simulink model "fftanalyzeri"  (R2012b)
settings: Solver=ode3  SolverMode=SingleTasking  StartTime=0.0  StopTime=20000  RelTol=1e-3
undefined symbols (not defined in the file or in its folder): pfb_coeff_gen_calc
undefined symbols (not defined in the file): fft_bin_flags_, magphmeanmem_, threshmem_
libraries: xbsIndex_r4 x9073, casper_library_misc x119, casper_library_flow_control x51, casper_library_delays x22, xps_library x10
(part 3 of 74)

== system fftanalyzeri/PulseDetector ==
  note: we take angle of 18.15. That is up to almost 4pi, or 4. normalixed by pi.
      | we want to nrmalize to +/-pi. So we keep buts 15 to 0, with bit 15 as a sign bit
      | This removes the 2pi jumps, keeping them around 0. We do not have
      | stuff around 2pi then stuff around 0-.
  note: Chan, din, dvldin can come on same clock.
      | we add puipe line delay for reading exp vals from the RAMs
  note: delauy for exp val ram read.
  note: Should be rams so we can save them...
  note: save current pylse bit, is_pulse, to ram, for this channel.
      | next time we read channel, we rememver if we are still reading a pulse
  note: Clear detected pulse
  note: rd en signal is a data valid signal, that will enable each part of the circult
  note: every time we switch which channel we are reading, we have to percuilate fresh data through this
      | whole circuit. it is 7 z's. so we have 7 clocks before we even know if there is a valid pulse or not.
      | The state machine controlling reading of the channel fifos must be able to wait for these 7 z's before it switches
      | to a new channel to read. We will generate a done sugnal telling that the pulse detection is done, and we are
      | free to readout a new channel fifo.
  note: rd signal aligend w/ output of pulse detector
  note: read sigakl delay- accounts for labntecy in the calcs
  note: 1 of pulse
      | 0 of no pulse
  note: Now we cpmpare  LLD with  the computed val
      | of 2 real samples, 2 im samples w/
      | DC offsets removed
  note: Add delayed sig w/ siang.
      | This does filtering by taking
      | two re samples and two im
      | samples and adding all
  note: Delay bu on sample
  note: Annd re and im together
  note: Take abs value to get all
      | piositive data
  note: Take out the expected value
      | or any DC offset
  note: delauy for exp val ram read.
  dvld_in : Inport
  din : Inport  Port=2
  clear : Inport  Port=3
  en : Inport  Port=4
  chan : Inport  Port=5
  savepulsestate : Inport  Port=6
  Absolute : xbsIndex_r4/Absolute  precision=User Defined  arith_type=Unsigned  n_bits=18  bin_pt=16  quantization=Truncate  overflow=Wrap  en=on  latency=1  dbl_ovrd=off  block_type=abs
  Absolute1 : xbsIndex_r4/Absolute  precision=User Defined  arith_type=Unsigned  n_bits=18  bin_pt=16  quantization=Truncate  overflow=Wrap  en=on  latency=1  dbl_ovrd=off  block_type=abs
  AddSub2 : xbsIndex_r4/AddSub  mode=Subtraction  use_carryin=off  use_carryout=off  en=on  latency=1  precision=User Defined  arith_type="Signed  (2's comp)"  n_bits=18  bin_pt=16  quantization=Truncate  overflow=Wrap  dbl_ovrd=off  use_behavioral_HDL=off  hw_selection=Fabric  pipelined=off  block_type=addsub
  AddSub3 : xbsIndex_r4/AddSub  mode=Subtraction  use_carryin=off  use_carryout=off  en=on  latency=1  precision=User Defined  arith_type="Signed  (2's comp)"  n_bits=18  bin_pt=16  quantization=Truncate  overflow=Wrap  dbl_ovrd=off  use_behavioral_HDL=off  hw_selection=Fabric  pipelined=off  block_type=addsub
  AddSub4 : xbsIndex_r4/AddSub  mode=Addition  use_carryin=off  use_carryout=off  en=on  latency=1  precision=User Defined  arith_type="Signed  (2's comp)"  n_bits=18  bin_pt=16  quantization=Truncate  overflow=Wrap  dbl_ovrd=off  use_behavioral_HDL=off  hw_selection=Fabric  pipelined=off  block_type=addsub
  AddSub5 : xbsIndex_r4/AddSub  mode=Addition  use_carryin=off  use_carryout=off  en=on  latency=1  precision=User Defined  arith_type="Signed  (2's comp)"  n_bits=19  bin_pt=16  quantization=Truncate  overflow=Wrap  dbl_ovrd=off  use_behavioral_HDL=off  hw_selection=Fabric  pipelined=off  block_type=addsub
  Delay{,6..8} (4 alike) : xbsIndex_r4/Delay  rst=on  infoeditControl=Selection of Reset will increase slice count due to use of real FFs and instead of SRLs  en=on  latency=1  dbl_ovrd=off  reg_retiming=off  block_type=delay
  Delay1 : xbsIndex_r4/Delay  rst=off  infoeditControl=Selection of Reset will increase slice count due to use of real FFs and instead of SRLs  en=on  latency=7  dbl_ovrd=off  reg_retiming=off  block_type=delay
  Delay2 : xbsIndex_r4/Delay  rst=on  infoeditControl=Selection of Reset will increase slice count due to use of real FFs and instead of SRLs  en=on  latency=5  dbl_ovrd=off  reg_retiming=off  block_type=delay
  Delay3 : xbsIndex_r4/Delay  rst=off  infoeditControl=Selection of Reset will increase slice count due to use of real FFs and instead of SRLs  en=on  latency=1  dbl_ovrd=off  reg_retiming=off  block_type=delay
  Delay4 : xbsIndex_r4/Delay  rst=off  infoeditControl=Selection of Reset will increase slice count due to use of real FFs and instead of SRLs  en=on  latency=1  dbl_ovrd=off  reg_retiming=off  block_type=delay
  Delay5 : xbsIndex_r4/Delay  rst=off  infoeditControl=Selection of Reset will increase slice count due to use of real FFs and instead of SRLs  en=off  latency=5  dbl_ovrd=off  reg_retiming=off  block_type=delay
  From Workspace2 : FromWorkspace  VariableName=PulseDetector_pulselength  SampleTime=1  Interpolate=off  OutputAfterFinalValue=Holding final value
  Gateway Out{,1..7} (8 alike) : xbsIndex_r4/Gateway Out  inherit_from_input=off  hdl_port=on  timing_constraint=None  locs_specified=off  LOCs={}  UseAsDAC=off  DACChannel='1'  block_type=gatewayout
  Logical : xbsIndex_r4/Logical  logical_function=OR  inputs=2  en=off  latency=0  precision=Full  arith_type=Unsigned  n_bits=16  bin_pt=0  align_bp=on  dbl_ovrd=off  block_type=logical
  Logical1 : xbsIndex_r4/Logical  logical_function=OR  inputs=2  en=off  latency=0  precision=Full  arith_type=Unsigned  n_bits=16  bin_pt=0  align_bp=on  dbl_ovrd=off  block_type=logical
  Logical{2..5} (4 alike) : xbsIndex_r4/Logical  logical_function=AND  inputs=2  en=off  latency=0  precision=Full  arith_type=Unsigned  n_bits=16  bin_pt=0  align_bp=on  dbl_ovrd=off  block_type=logical
  Normalize180_ : Subsystem
  Normalize180_1 : Subsystem
  PulseLenCounter : xbsIndex_r4/Counter  cnt_type=Free Running  cnt_to=0  operation=Down  start_count=0  cnt_by_val=1  arith_type=Unsigned  n_bits=8  bin_pt=0  load_pin=on  rst=on  en=on  explicit_period=on  period=1  dbl_ovrd=off  use_behavioral_HDL=off  implementation=Fabric  block_type=counter
  PulseLength : xbsIndex_r4/Register  init=0  rst=on  en=on  dbl_ovrd=off  block_type=register
  Register1 : xbsIndex_r4/Register  init=0  rst=off  en=on  dbl_ovrd=off  block_type=register
  Relational : xbsIndex_r4/Relational  mode=a>b  en=off  latency=0  dbl_ovrd=off  block_type=relational
  Relational1 : xbsIndex_r4/Relational  mode=a!=b  en=off  latency=0  dbl_ovrd=off  block_type=relational
  bits_31_16_ : xbsIndex_r4/Slice  nbits=16  boolean_output=off  mode=Lower Bit Location + Width  bit1=0  base1=MSB of Input  bit0=16  base0=LSB of Input  dbl_ovrd=off  block_type=slice
  bool_ : xbsIndex_r4/Constant  const=0  gui_display_data_type=Boolean  arith_type=Boolean  n_bits=16  bin_pt=14  preci_type=Single  exp_width=8  frac_width=24  explicit_period=on  period=1  equ=P=C  opselect=C  inp2=PCIN>>17  opr=+  inp1=P  carry=CIN  dbl_ovrd=off  block_type=constant
  bool_6 : xbsIndex_r4/Constant  const=0  gui_display_data_type=Boolean  arith_type=Boolean  n_bits=16  bin_pt=14  preci_type=Single  exp_width=8  frac_width=24  explicit_period=on  period=1  equ=P=C  opselect=C  inp2=PCIN>>17  opr=+  inp1=P  carry=CIN  dbl_ovrd=off  block_type=constant
  bool_7 : xbsIndex_r4/Constant  const=1  gui_display_data_type=Boolean  arith_type=Boolean  n_bits=16  bin_pt=14  preci_type=Single  exp_width=8  frac_width=24  explicit_period=on  period=1  equ=P=C  opselect=C  inp2=PCIN>>17  opr=+  inp1=P  carry=CIN  dbl_ovrd=off  block_type=constant
  buts_15_0_ : xbsIndex_r4/Slice  nbits=16  boolean_output=off  mode=Lower Bit Location + Width  bit1=0  base1=MSB of Input  bit0=0  base0=LSB of Input  dbl_ovrd=off  block_type=slice
  buts_17_0_ : xbsIndex_r4/Slice  nbits=18  boolean_output=off  mode=Lower Bit Location + Width  bit1=0  base1=MSB of Input  bit0=0  base0=LSB of Input  dbl_ovrd=off  block_type=slice
  buts_7_0_1 : xbsIndex_r4/Slice  nbits=8  boolean_output=off  mode=Lower Bit Location + Width  bit1=0  base1=MSB of Input  bit0=0  base0=LSB of Input  dbl_ovrd=off  block_type=slice
  c2polar_ : Subsystem
  i16_13_2 : xbsIndex_r4/Reinterpret  force_arith_type=on  arith_type="Signed  (2's comp)"  force_bin_pt=on  bin_pt=13  block_type=reinterpret
  i16_14_1 : xbsIndex_r4/Reinterpret  force_arith_type=on  arith_type="Signed  (2's comp)"  force_bin_pt=on  bin_pt=14  block_type=reinterpret
  i18_16_3 : xbsIndex_r4/Reinterpret  force_arith_type=on  arith_type="Signed  (2's comp)"  force_bin_pt=on  bin_pt=16  block_type=reinterpret
  lsb8_ : xbsIndex_r4/Slice  nbits=8  boolean_output=off  mode=Lower Bit Location + Width  bit1=0  base1=MSB of Input  bit0=0  base0=LSB of Input  dbl_ovrd=off  block_type=slice
  meanmagph32_ : Subsystem  Tag=xps:bram  AncestorBlock=xps_library/Shared BRAM  mask{arith_type=Unsigned, addr_width=10, data_width=32, reg_prim_output=off, reg_core_output=off, optimization=Minimum_Area, data_bin_pt=0, init_vals=magphmeanmem_, sample_rate=1}
      mask prompts: arith_type "Output Data Type"; addr_width "Address width"; data_width "Data Width"; reg_prim_output "Register Primitive Output"; reg_core_output "Register Core Output"; data_bin_pt "Data Binary Point"; init_vals "Initial values (simulation only)"; sample_rate "Sample rate"
      mask init:
      | shared_bram_mask;
      mask TypeOptions arith_type: Unsigned | Signed  (2's comp)
      mask TypeOptions data_width: 8 | 16 | 32 | 64 | 128
      mask TypeOptions optimization: Minimum_Area | Low_Power
  pulseDetScope : Scope  NumInputPorts=8
      settings: YMin=-5~-5~-5~-5~-5~-5~-5~-5  YMax=5~5~5~5~5~5~5~5  SaveName=fsmdata2
  pulselength : Subsystem  Tag=xps:sw_reg  AncestorBlock=xps_library/software register  mask{numios=1, io_dir=From Processor, io_delay=0, sample_period=1, name1=reg, bitwidth1=32, arith_type1=Unsigned, bin_pt1=0}
      mask prompts: numios "Num I/Os"; io_dir "I/O direction"; io_delay "I/O delay"; sample_period "Sample period"; name1 "Name"; bitwidth1 "Bitwidth"; arith_type1 "Type"; bin_pt1 "Binary pt"
      mask init:
      | swreg_init(gcb);
      mask Callback numios: t = timer('StartDelay', 0.1); t.TimerFcn = {@swreg_cb, gcb}; start(t);
      mask TypeOptions io_dir: To Processor | From Processor
      mask Callback io_dir:
      | a = get_param(gcb, 'MaskEnables');
      | if strcmp(get_param(gcb, 'io_dir'), 'To Processor'),
      | a(4) = {'off'};
      | else
      | a(4) = {'on'};
      | end
      | set_param(gcb, 'MaskEnables', a);
      mask TypeOptions arith_type1: Unsigned | Signed  (2's comp) | Boolean
      mask Callback arith_type1:
      | a = get_param(gcb, 'MaskEnables');
      | if strcmp(get_param(gcb, 'arith_type1'), 'Boolean'),
      | set_param(gcb, 'bitwidth1', '1');
      | set_param(gcb, 'bin_pt1', '0');
      | a(6) = {'off'};
      | a(8) = {'off'};
      | else
      | a(6) = {'on'};
      | a(8) = {'on'};
      | end
      | set_param(gcb, 'MaskEnables', a);
  pulsestateRAM : xbsIndex_r4/Single Port RAM  depth=256  initVector=zeros(1,256)  distributed_mem=Block RAM  write_mode=Read After Write  rst=off  init_reg=0  en=off  latency=1  dbl_ovrd=off  optimize=Area  use_rpm=on  block_type=spram
  thresh32_1 : Subsystem  Tag=xps:bram  AncestorBlock=xps_library/Shared BRAM  mask{arith_type=Unsigned, addr_width=10, data_width=32, reg_prim_output=off, reg_core_output=off, optimization=Minimum_Area, data_bin_pt=0, init_vals=threshmem_, sample_rate=1}
      mask prompts: arith_type "Output Data Type"; addr_width "Address width"; data_width "Data Width"; reg_prim_output "Register Primitive Output"; reg_core_output "Register Core Output"; data_bin_pt "Data Binary Point"; init_vals "Initial values (simulation only)"; sample_rate "Sample rate"
      mask init:
      | shared_bram_mask;
      mask TypeOptions arith_type: Unsigned | Signed  (2's comp)
      mask TypeOptions data_width: 8 | 16 | 32 | 64 | 128
      mask TypeOptions optimization: Minimum_Area | Low_Power
  ui8_1 : xbsIndex_r4/Constant  const=0  gui_display_data_type=Fixed-point  arith_type=Unsigned  n_bits=8  bin_pt=0  preci_type=Single  exp_width=8  frac_width=24  explicit_period=on  period=1  equ=P=C  opselect=C  inp2=PCIN>>17  opr=+  inp1=P  carry=CIN  dbl_ovrd=off  block_type=constant
  uint32_ : xbsIndex_r4/Constant  const=0  gui_display_data_type=Fixed-point  arith_type=Unsigned  n_bits=32  bin_pt=0  preci_type=Single  exp_width=8  frac_width=24  explicit_period=on  period=1  equ=P=C  opselect=C  inp2=PCIN>>17  opr=+  inp1=P  carry=CIN  dbl_ovrd=off  block_type=constant
  datadly : Outport
  dvld_out : Outport  Port=2
  busy : Outport  Port=3
  pulse : Outport  Port=4
  detect : Outport  Port=5
  savedpulsestate : Outport  Port=6
  wires:
  Register1/1 -> AddSub5/2
  [magExpVal] -> AddSub2/2
  [phaseExpVal] -> Gateway Out2/1, AddSub3/2
  Delay8/1 -> detect/1, Logical/1, PulseLenCounter/1, Gateway Out7/1
  AddSub2/1 -> Absolute/1
  ui8_1/1 -> Relational1/1
  din/1 -> c2polar_/1(c), Delay1/1
  Absolute/1 -> AddSub4/1
  AddSub3/1 -> Normalize180_1/1(In1), Gateway Out3/1
  Absolute1/1 -> AddSub4/2, Gateway Out4/1
  Delay/1 -> Logical4/1, dvld_out/1, Logical1/1
  AddSub4/1 -> Gateway Out5/1, AddSub5/1, Register1/1
  PulseLenCounter/1 -> Relational1/2
  bool_7/1 -> PulseLength/3
  Delay5/1 -> Relational/2
  Delay1/1 -> datadly/1
  dvld_in/1 -> Delay2/1
  Relational1/1 -> Logical/2, Delay7/1
  bool_6/1 -> PulseLength/2
  AddSub5/1 -> Gateway Out6/1, Relational/1
  [pls_thresh] -> Delay5/1
  Logical1/1 -> busy/1
  Delay6/1 -> Logical2/1, Delay/1
  clear/1 -> Delay2/2, Delay/2, Delay6/2, Delay8/2, PulseLenCounter/3, Delay7/2
  Delay7/1 -> [is_pulse], pulse/1, Logical1/2
  Relational/1 -> Delay8/1
  PulseLength/1 -> PulseLenCounter/2
  en/1 -> [enable]
  [enable] -> Delay3/2, Delay2/3, Delay1/2, Delay/3, Delay6/3
  [enable] -> AddSub4/3, Absolute/2, Absolute1/2, AddSub2/3, AddSub3/3
  [enable] -> Register1/2
  Logical2/1 -> Delay8/3
  [enable] -> Logical2/2
  Logical3/1 -> PulseLenCounter/4
  Logical/1 -> Logical3/1
  [enable] -> Logical3/2
  Logical4/1 -> Delay7/3
  [enable] -> Logical4/2
  Delay2/1 -> Logical5/1, Delay6/1
  [enable] -> Logical5/2
  Logical5/1 -> AddSub5/3
  savepulsestate/1 -> pulsestateRAM/3
  [is_pulse] -> pulsestateRAM/2
  pulsestateRAM/1 -> savedpulsestate/1
  Delay3/1 -> AddSub2/1
  Delay4/1 -> Gateway Out1/1, AddSub3/1
  [enable] -> Delay4/2
  lsb8_/1 -> thresh32_1/1(addr), meanmagph32_/1(addr), pulsestateRAM/1
  c2polar_/2(phase) -> Gateway Out/1, Normalize180_/1(In1)
  c2polar_/1(power) -> Delay3/1
  pulselength/1(in_reg) -> buts_7_0_1/1
  From Workspace2/1 -> pulselength/1(sim_reg)
  buts_7_0_1/1 -> [pls_len]
  [pls_len] -> PulseLength/1
  Gateway Out/1 -> pulseDetScope/1
  Gateway Out1/1 -> pulseDetScope/2
  Gateway Out2/1 -> pulseDetScope/3
  Gateway Out3/1 -> pulseDetScope/4
  Gateway Out4/1 -> pulseDetScope/5
  Gateway Out5/1 -> pulseDetScope/6
  Gateway Out6/1 -> pulseDetScope/7
  Gateway Out7/1 -> pulseDetScope/8
  chan/1 -> lsb8_/1
  buts_15_0_/1 -> i16_14_1/1
  bits_31_16_/1 -> i16_13_2/1
  buts_17_0_/1 -> i18_16_3/1
  i16_14_1/1 -> [magExpVal]
  i16_13_2/1 -> [phaseExpVal]
  meanmagph32_/1(data_out) -> buts_15_0_/1, bits_31_16_/1
  i18_16_3/1 -> [pls_thresh]
  bool_/1 -> thresh32_1/3(we), meanmagph32_/3(we)
  thresh32_1/1(data_out) -> buts_17_0_/1
  uint32_/1 -> thresh32_1/2(data_in), meanmagph32_/2(data_in)
  Normalize180_/1(Out1) -> Delay4/1
  Normalize180_1/1(Out1) -> Absolute1/1

== system fftanalyzeri/RWen ==
  sim_reg : Inport
  fftanalyzeri_RWen_user_data_out : xbsIndex_r4/Gateway In  gui_display_data_type=Fixed-point  arith_type=Unsigned  n_bits=32  bin_pt=0  preci_type=Single  exp_width=8  frac_width=24  quantization="Round  (unbiased: +/- Inf)"  overflow=Saturate  period=1  dbl_ovrd=off  timing_constraint=None  locs_specified=off  LOCs={}  UseAsADC=off  ADCChannel='1'  inherit_from_input=off  hdl_port=on  block_type=gatewayin
  io_delay : xbsIndex_r4/Delay  rst=off  infoeditControl=Selection of Reset will increase slice count due to use of real FFs and instead of SRLs  en=off  latency=0  dbl_ovrd=off  reg_retiming=on  block_type=delay
  reint1 : xbsIndex_r4/Reinterpret  force_arith_type=on  arith_type=Unsigned  force_bin_pt=on  bin_pt=0  block_type=reinterpret
  slice_reg : xbsIndex_r4/Slice  nbits=32  boolean_output=off  mode=Lower Bit Location + Width  bit1=0  base1=MSB of Input  bit0=0  base0=LSB of Input  dbl_ovrd=off  block_type=slice
  in_reg : Outport
  wires:
  fftanalyzeri_RWen_user_data_out/1 -> io_delay/1
  sim_reg/1 -> fftanalyzeri_RWen_user_data_out/1
  io_delay/1 -> slice_reg/1
  slice_reg/1 -> reint1/1
  reint1/1 -> in_reg/1

== system fftanalyzeri/RectToPolar ==
  note: shoudl be same delay as cordic. if it takes 18 clocks to go
      | through cordic, it hould be 18 here.
  note: input re and im.
      | output magnitude and phase
      | phase is from 0 to 2, where 2 is 2pi.
      | put as complex number where im part is actuaol phase
      | 18 bit data, phase in NOT radians but mult of pi.
      | phse/pi is output. Translate alg. where imagine we translate the vector (k,0)
      | phase is how much we rotated the cord. to make the 0.
  dvld_in : Inport
  cmplx_din : Inport  Port=2
  chan : Inport  Port=3
  "CORDIC 4.0 " : xbsIndex_r4/CORDIC 4.0   functional_selection=Translate  architectural_configuration=Parallel  pipelining_mode=Maximum  data_format=SignedFraction  phase_format=Scaled_Radians  output_width=18  round_mode=Truncate  iterations=0  precision=0  coarse_rotation=on  compensation_scaling=Embedded_Multiplier  ce=off  sclr=off  nd=on  rdy=on  x_out=on  y_out=off  phase_output=on  register_inputs=true  register_outputs=true  ipcore_usecache=true  ipcore_useipmodelcache=true  ipcore_verbose=false  wrapper_available=true  ip_name=CORDIC  ip_version=4.0  dsptool_ready=true  port_translation_map={ 'ce' => 'en', 'sclr' => 'rst' }  structural_sim=false  block_type=cordic_v4_0
  Delay : xbsIndex_r4/Delay  rst=off  infoeditControl=Selection of Reset will increase slice count due to use of real FFs and instead of SRLs  en=off  latency=25  dbl_ovrd=off  reg_retiming=off  block_type=delay
  Gateway Out{1..4,34..37} (8 alike) : xbsIndex_r4/Gateway Out  inherit_from_input=off  hdl_port=on  timing_constraint=None  locs_specified=off  LOCs={}  UseAsDAC=off  DACChannel='1'  block_type=gatewayout
  c_to_ri3 : casper_library_misc/c_to_ri  n_bits=18  bin_pt=16
      settings: AttributesFormatString=18_16 r/i
  i18_16_1 : xbsIndex_r4/Assert  assert_type=on  type_source=Explicitly  gui_display_data_type=Fixed-point  arith_type="Signed  (2's comp)"  n_bits=18  bin_pt=16  preci_type=Single  exp_width=8  frac_width=24  assert_rate=off  rate_source=Explicitly  period=1  output_port=on  block_type=assert
  i18_16_2 : xbsIndex_r4/Assert  assert_type=on  type_source=Explicitly  gui_display_data_type=Fixed-point  arith_type="Signed  (2's comp)"  n_bits=18  bin_pt=16  preci_type=Single  exp_width=8  frac_width=24  assert_rate=off  rate_source=Explicitly  period=1  output_port=on  block_type=assert
  rect2polar : Scope  NumInputPorts=8
      settings: YMin=-5~-5~-5~-5~-5~-5~-5~-5  YMax=5~5~5~5~5~5~5~5  SaveName=fsmdata10
  ri_to_c : casper_library_misc/ri_to_c
  dvld_out : Outport
  cmplx_dout : Outport  Port=2
  chandly : Outport  Port=3
  wires:
  c_to_ri3/2 -> Gateway Out37/1, i18_16_1/1
  dvld_in/1 -> Gateway Out3/1, "CORDIC 4.0 "/3
  c_to_ri3/1 -> Gateway Out36/1, i18_16_2/1
  ri_to_c/1 -> cmplx_dout/1
  "CORDIC 4.0 "/3 -> Gateway Out4/1, dvld_out/1
  "CORDIC 4.0 "/1 -> Gateway Out34/1, ri_to_c/1
  "CORDIC 4.0 "/2 -> Gateway Out35/1, ri_to_c/2
  i18_16_2/1 -> "CORDIC 4.0 "/1
  i18_16_1/1 -> "CORDIC 4.0 "/2
  cmplx_din/1 -> c_to_ri3/1
  Delay/1 -> Gateway Out2/1, chandly/1
  chan/1 -> Gateway Out1/1, Delay/1
  Gateway Out36/1 -> rect2polar/1
  Gateway Out37/1 -> rect2polar/2
  Gateway Out34/1 -> rect2polar/3
  Gateway Out35/1 -> rect2polar/4
  Gateway Out3/1 -> rect2polar/5
  Gateway Out4/1 -> rect2polar/6
  Gateway Out1/1 -> rect2polar/7
  Gateway Out2/1 -> rect2polar/8

== system fftanalyzeri/RectToPolar1 ==
  note: shoudl be same delay as cordic. if it takes 18 clocks to go
      | through cordic, it hould be 18 here.
  note: input re and im.
      | output magnitude and phase
      | phase is from 0 to 2, where 2 is 2pi.
      | put as complex number where im part is actuaol phase
      | 18 bit data, phase in NOT radians but mult of pi.
      | phse/pi is output. Translate alg. where imagine we translate the vector (k,0)
      | phase is how much we rotated the cord. to make the 0.
  dvld_in : Inport
  cmplx_din : Inport  Port=2
  chan : Inport  Port=3
  "CORDIC 4.0 " : xbsIndex_r4/CORDIC 4.0   functional_selection=Translate  architectural_configuration=Parallel  pipelining_mode=Maximum  data_format=SignedFraction  phase_format=Scaled_Radians  output_width=18  round_mode=Truncate  iterations=0  precision=0  coarse_rotation=on  compensation_scaling=Embedded_Multiplier  ce=off  sclr=off  nd=on  rdy=on  x_out=on  y_out=off  phase_output=on  register_inputs=true  register_outputs=true  ipcore_usecache=true  ipcore_useipmodelcache=true  ipcore_verbose=false  wrapper_available=true  ip_name=CORDIC  ip_version=4.0  dsptool_ready=true  port_translation_map={ 'ce' => 'en', 'sclr' => 'rst' }  structural_sim=false  block_type=cordic_v4_0
  Delay : xbsIndex_r4/Delay  rst=off  infoeditControl=Selection of Reset will increase slice count due to use of real FFs and instead of SRLs  en=off  latency=25  dbl_ovrd=off  reg_retiming=off  block_type=delay
  c_to_ri3 : casper_library_misc/c_to_ri  n_bits=18  bin_pt=16
      settings: AttributesFormatString=18_16 r/i
  i18_16_1 : xbsIndex_r4/Assert  assert_type=on  type_source=Explicitly  gui_display_data_type=Fixed-point  arith_type="Signed  (2's comp)"  n_bits=18  bin_pt=16  preci_type=Single  exp_width=8  frac_width=24  assert_rate=off  rate_source=Explicitly  period=1  output_port=on  block_type=assert
  i18_16_2 : xbsIndex_r4/Assert  assert_type=on  type_source=Explicitly  gui_display_data_type=Fixed-point  arith_type="Signed  (2's comp)"  n_bits=18  bin_pt=16  preci_type=Single  exp_width=8  frac_width=24  assert_rate=off  rate_source=Explicitly  period=1  output_port=on  block_type=assert
  ri_to_c : casper_library_misc/ri_to_c
  dvld_out : Outport
  cmplx_dout : Outport  Port=2
  chandly : Outport  Port=3
  wires:
  c_to_ri3/2 -> i18_16_1/1
  dvld_in/1 -> "CORDIC 4.0 "/3
  c_to_ri3/1 -> i18_16_2/1
  ri_to_c/1 -> cmplx_dout/1
  "CORDIC 4.0 "/3 -> dvld_out/1
  "CORDIC 4.0 "/1 -> ri_to_c/1
  "CORDIC 4.0 "/2 -> ri_to_c/2
  i18_16_2/1 -> "CORDIC 4.0 "/1
  i18_16_1/1 -> "CORDIC 4.0 "/2
  cmplx_din/1 -> c_to_ri3/1
  Delay/1 -> chandly/1
  chan/1 -> Delay/1

== system fftanalyzeri/RectToPolar2 ==
  note: shoudl be same delay as cordic. if it takes 18 clocks to go
      | through cordic, it hould be 18 here.
  note: input re and im.
      | output magnitude and phase
      | phase is from 0 to 2, where 2 is 2pi.
      | put as complex number where im part is actuaol phase
      | 18 bit data, phase in NOT radians but mult of pi.
      | phse/pi is output. Translate alg. where imagine we translate the vector (k,0)
      | phase is how much we rotated the cord. to make the 0.
  dvld_in : Inport
  cmplx_din : Inport  Port=2
  chan : Inport  Port=3
  "CORDIC 4.0 " : xbsIndex_r4/CORDIC 4.0   functional_selection=Translate  architectural_configuration=Parallel  pipelining_mode=Maximum  data_format=SignedFraction  phase_format=Scaled_Radians  output_width=18  round_mode=Truncate  iterations=0  precision=0  coarse_rotation=on  compensation_scaling=Embedded_Multiplier  ce=off  sclr=off  nd=on  rdy=on  x_out=on  y_out=off  phase_output=on  register_inputs=true  register_outputs=true  ipcore_usecache=true  ipcore_useipmodelcache=true  ipcore_verbose=false  wrapper_available=true  ip_name=CORDIC  ip_version=4.0  dsptool_ready=true  port_translation_map={ 'ce' => 'en', 'sclr' => 'rst' }  structural_sim=false  block_type=cordic_v4_0
  Delay : xbsIndex_r4/Delay  rst=off  infoeditControl=Selection of Reset will increase slice count due to use of real FFs and instead of SRLs  en=off  latency=25  dbl_ovrd=off  reg_retiming=off  block_type=delay
  c_to_ri3 : casper_library_misc/c_to_ri  n_bits=18  bin_pt=16
      settings: AttributesFormatString=18_16 r/i
  i18_16_1 : xbsIndex_r4/Assert  assert_type=on  type_source=Explicitly  gui_display_data_type=Fixed-point  arith_type="Signed  (2's comp)"  n_bits=18  bin_pt=16  preci_type=Single  exp_width=8  frac_width=24  assert_rate=off  rate_source=Explicitly  period=1  output_port=on  block_type=assert
  i18_16_2 : xbsIndex_r4/Assert  assert_type=on  type_source=Explicitly  gui_display_data_type=Fixed-point  arith_type="Signed  (2's comp)"  n_bits=18  bin_pt=16  preci_type=Single  exp_width=8  frac_width=24  assert_rate=off  rate_source=Explicitly  period=1  output_port=on  block_type=assert
  ri_to_c : casper_library_misc/ri_to_c
  dvld_out : Outport
  cmplx_dout : Outport  Port=2
  chandly : Outport  Port=3
  wires:
  c_to_ri3/2 -> i18_16_1/1
  dvld_in/1 -> "CORDIC 4.0 "/3
  c_to_ri3/1 -> i18_16_2/1
  ri_to_c/1 -> cmplx_dout/1
  "CORDIC 4.0 "/3 -> dvld_out/1
  "CORDIC 4.0 "/1 -> ri_to_c/1
  "CORDIC 4.0 "/2 -> ri_to_c/2
  i18_16_2/1 -> "CORDIC 4.0 "/1
  i18_16_1/1 -> "CORDIC 4.0 "/2
  cmplx_din/1 -> c_to_ri3/1
  Delay/1 -> chandly/1
  chan/1 -> Delay/1

== system fftanalyzeri/RectToPolar3 ==
  note: shoudl be same delay as cordic. if it takes 18 clocks to go
      | through cordic, it hould be 18 here.
  note: input re and im.
      | output magnitude and phase
      | phase is from 0 to 2, where 2 is 2pi.
      | put as complex number where im part is actuaol phase
      | 18 bit data, phase in NOT radians but mult of pi.
      | phse/pi is output. Translate alg. where imagine we translate the vector (k,0)
      | phase is how much we rotated the cord. to make the 0.
  dvld_in : Inport
  cmplx_din : Inport  Port=2
  chan : Inport  Port=3
  "CORDIC 4.0 " : xbsIndex_r4/CORDIC 4.0   functional_selection=Translate  architectural_configuration=Parallel  pipelining_mode=Maximum  data_format=SignedFraction  phase_format=Scaled_Radians  output_width=18  round_mode=Truncate  iterations=0  precision=0  coarse_rotation=on  compensation_scaling=Embedded_Multiplier  ce=off  sclr=off  nd=on  rdy=on  x_out=on  y_out=off  phase_output=on  register_inputs=true  register_outputs=true  ipcore_usecache=true  ipcore_useipmodelcache=true  ipcore_verbose=false  wrapper_available=true  ip_name=CORDIC  ip_version=4.0  dsptool_ready=true  port_translation_map={ 'ce' => 'en', 'sclr' => 'rst' }  structural_sim=false  block_type=cordic_v4_0
  Delay : xbsIndex_r4/Delay  rst=off  infoeditControl=Selection of Reset will increase slice count due to use of real FFs and instead of SRLs  en=off  latency=25  dbl_ovrd=off  reg_retiming=off  block_type=delay
  c_to_ri3 : casper_library_misc/c_to_ri  n_bits=18  bin_pt=16
      settings: AttributesFormatString=18_16 r/i
  i18_16_1 : xbsIndex_r4/Assert  assert_type=on  type_source=Explicitly  gui_display_data_type=Fixed-point  arith_type="Signed  (2's comp)"  n_bits=18  bin_pt=16  preci_type=Single  exp_width=8  frac_width=24  assert_rate=off  rate_source=Explicitly  period=1  output_port=on  block_type=assert
  i18_16_2 : xbsIndex_r4/Assert  assert_type=on  type_source=Explicitly  gui_display_data_type=Fixed-point  arith_type="Signed  (2's comp)"  n_bits=18  bin_pt=16  preci_type=Single  exp_width=8  frac_width=24  assert_rate=off  rate_source=Explicitly  period=1  output_port=on  block_type=assert
  ri_to_c : casper_library_misc/ri_to_c
  dvld_out : Outport
  cmplx_dout : Outport  Port=2
  chandly : Outport  Port=3
  wires:
  c_to_ri3/2 -> i18_16_1/1
  dvld_in/1 -> "CORDIC 4.0 "/3
  c_to_ri3/1 -> i18_16_2/1
  ri_to_c/1 -> cmplx_dout/1
  "CORDIC 4.0 "/3 -> dvld_out/1
  "CORDIC 4.0 "/1 -> ri_to_c/1
  "CORDIC 4.0 "/2 -> ri_to_c/2
  i18_16_2/1 -> "CORDIC 4.0 "/1
  i18_16_1/1 -> "CORDIC 4.0 "/2
  cmplx_din/1 -> c_to_ri3/1
  Delay/1 -> chandly/1
  chan/1 -> Delay/1

== system fftanalyzeri/SER_DI ==
  sim_reg : Inport
  fftanalyzeri_SER_DI_user_data_out : xbsIndex_r4/Gateway In  gui_display_data_type=Fixed-point  arith_type=Unsigned  n_bits=32  bin_pt=0  preci_type=Single  exp_width=8  frac_width=24  quantization="Round  (unbiased: +/- Inf)"  overflow=Saturate  period=1  dbl_ovrd=off  timing_constraint=None  locs_specified=off  LOCs={}  UseAsADC=off  ADCChannel='1'  inherit_from_input=off  hdl_port=on  block_type=gatewayin
  io_delay : xbsIndex_r4/Delay  rst=off  infoeditControl=Selection of Reset will increase slice count due to use of real FFs and instead of SRLs  en=off  latency=0  dbl_ovrd=off  reg_retiming=on  block_type=delay
  reint1 : xbsIndex_r4/Reinterpret  force_arith_type=on  arith_type=Unsigned  force_bin_pt=on  bin_pt=0  block_type=reinterpret
  slice_reg : xbsIndex_r4/Slice  nbits=32  boolean_output=off  mode=Lower Bit Location + Width  bit1=0  base1=MSB of Input  bit0=0  base0=LSB of Input  dbl_ovrd=off  block_type=slice
  in_reg : Outport
  wires:
  fftanalyzeri_SER_DI_user_data_out/1 -> io_delay/1
  sim_reg/1 -> fftanalyzeri_SER_DI_user_data_out/1
  io_delay/1 -> slice_reg/1
  slice_reg/1 -> reint1/1
  reint1/1 -> in_reg/1

== system fftanalyzeri/SWAT_LE ==
  sim_reg : Inport
  fftanalyzeri_SWAT_LE_user_data_out : xbsIndex_r4/Gateway In  gui_display_data_type=Fixed-point  arith_type=Unsigned  n_bits=32  bin_pt=0  preci_type=Single  exp_width=8  frac_width=24  quantization="Round  (unbiased: +/- Inf)"  overflow=Saturate  period=1  dbl_ovrd=off  timing_constraint=None  locs_specified=off  LOCs={}  UseAsADC=off  ADCChannel='1'  inherit_from_input=off  hdl_port=on  block_type=gatewayin
  io_delay : xbsIndex_r4/Delay  rst=off  infoeditControl=Selection of Reset will increase slice count due to use of real FFs and instead of SRLs  en=off  latency=0  dbl_ovrd=off  reg_retiming=on  block_type=delay
  reint1 : xbsIndex_r4/Reinterpret  force_arith_type=on  arith_type=Unsigned  force_bin_pt=on  bin_pt=0  block_type=reinterpret
  slice_reg : xbsIndex_r4/Slice  nbits=32  boolean_output=off  mode=Lower Bit Location + Width  bit1=0  base1=MSB of Input  bit0=0  base0=LSB of Input  dbl_ovrd=off  block_type=slice
  in_reg : Outport
  wires:
  fftanalyzeri_SWAT_LE_user_data_out/1 -> io_delay/1
  sim_reg/1 -> fftanalyzeri_SWAT_LE_user_data_out/1
  io_delay/1 -> slice_reg/1
  slice_reg/1 -> reint1/1
  reint1/1 -> in_reg/1

== system fftanalyzeri/adcWaveMem ==
  Start : Inport
  Sel : Inport  Port=2
  Src0 : Inport  Port=3
  Src1 : Inport  Port=4
  WE : Inport  Port=5
  WE1 : Inport  Port=6
  Logical : xbsIndex_r4/Logical  logical_function=OR  inputs=2  en=off  latency=0  precision=Full  arith_type=Unsigned  n_bits=16  bin_pt=0  align_bp=on  dbl_ovrd=off  block_type=logical
  MemRecord : Subsystem
  Mux : xbsIndex_r4/Mux  inputs=2  en=off  latency=0  precision=Full  arith_type=Unsigned  n_bits=16  bin_pt=14  quantization=Truncate  overflow=Wrap  dbl_ovrd=off  block_type=mux
  Slice : xbsIndex_r4/Slice  nbits=12  boolean_output=off  mode=Lower Bit Location + Width  bit1=0  base1=LSB of Input  bit0=0  base0=LSB of Input  dbl_ovrd=off  block_type=slice
  edge_detect : casper_library_misc/edge_detect  edge=Rising  polarity=Active High  x_in=[0 0.08 0.08 0.16 0.16 0.24 0.24 0.32 0.32 0.4]  y_in="[-1 -1  1  1  1  1  1  1  1  1]"  x_out=[0.6 0.68 0.68 0.76 0.76 0.84 0.84 0.92 0.92 1]  y_out="[-1 -1  1  1 -1 -1 -1 -1 -1 -1]"
  Out1 : Outport
  wires:
  Sel/1 -> Mux/1
  edge_detect/1 -> Logical/2
  WE/1 -> Logical/1
  Src0/1 -> Mux/2
  Src1/1 -> Mux/3
  WE1/1 -> edge_detect/1
  MemRecord/1(memDone) -> Out1/1
  Start/1 -> MemRecord/1(Start)
  Logical/1 -> MemRecord/3(WE)
  Slice/1 -> MemRecord/2(DataIn)
  Mux/1 -> Slice/1

== system fftanalyzeri/bincount_out ==
  out_reg : Inport
  cast_gw : xbsIndex_r4/Convert  gui_display_data_type=Fixed-point  arith_type=Unsigned  n_bits=32  bin_pt=0  float_type=Single  exp_bits=8  fraction_bits=24  quantization=Truncate  overflow=Wrap  en=off  latency=0  dbl_ovrd=off  pipeline=off  block_type=convert
  fftanalyzeri_bincount_out_user_data_in : xbsIndex_r4/Gateway Out  inherit_from_input=off  hdl_port=on  timing_constraint=None  locs_specified=off  LOCs={}  UseAsDAC=off  DACChannel='1'  block_type=gatewayout
  io_delay : xbsIndex_r4/Delay  rst=off  infoeditControl=Selection of Reset will increase slice count due to use of real FFs and instead of SRLs  en=off  latency=0  dbl_ovrd=off  reg_retiming=on  block_type=delay
  reint1 : xbsIndex_r4/Reinterpret  force_arith_type=on  arith_type=Unsigned  force_bin_pt=on  bin_pt=0  block_type=reinterpret
  sim_out : Outport
  wires:
  io_delay/1 -> cast_gw/1
  cast_gw/1 -> fftanalyzeri_bincount_out_user_data_in/1
  fftanalyzeri_bincount_out_user_data_in/1 -> sim_out/1
  out_reg/1 -> reint1/1
  reint1/1 -> io_delay/1

== system fftanalyzeri/c2Polar16_2 ==
  c : Inport
  b17_2_ : xbsIndex_r4/Slice  nbits=16  boolean_output=off  mode=Lower Bit Location + Width  bit1=0  base1=MSB of Input  bit0=0  base0=LSB of Input  dbl_ovrd=off  block_type=slice
  b33_16_ : xbsIndex_r4/Slice  nbits=16  boolean_output=off  mode=Lower Bit Location + Width  bit1=2  base1=MSB of Input  bit0=16  base0=LSB of Input  dbl_ovrd=off  block_type=slice
  i16_13 : xbsIndex_r4/Reinterpret  force_arith_type=on  arith_type="Signed  (2's comp)"  force_bin_pt=on  bin_pt=13  block_type=reinterpret
  ui16_16_ : xbsIndex_r4/Reinterpret  force_arith_type=on  arith_type=Unsigned  force_bin_pt=on  bin_pt=16  block_type=reinterpret
  power : Outport
  phase : Outport  Port=2
  wires:
  i16_13/1 -> phase/1
  c/1 -> b17_2_/1, b33_16_/1
  ui16_16_/1 -> power/1
  b33_16_/1 -> ui16_16_/1
  b17_2_/1 -> i16_13/1

== system fftanalyzeri/c2TruncatePolar16_1 ==
  c : Inport
  b17_2_ : xbsIndex_r4/Slice  nbits=16  boolean_output=off  mode=Lower Bit Location + Width  bit1=0  base1=MSB of Input  bit0=2  base0=LSB of Input  dbl_ovrd=off  block_type=slice
  b33_16_ : xbsIndex_r4/Slice  nbits=16  boolean_output=off  mode=Lower Bit Location + Width  bit1=2  base1=MSB of Input  bit0=18  base0=LSB of Input  dbl_ovrd=off  block_type=slice
  i16_13 : xbsIndex_r4/Reinterpret  force_arith_type=on  arith_type="Signed  (2's comp)"  force_bin_pt=on  bin_pt=13  block_type=reinterpret
  ui16_16_ : xbsIndex_r4/Reinterpret  force_arith_type=on  arith_type=Unsigned  force_bin_pt=on  bin_pt=16  block_type=reinterpret
  power : Outport
  phase : Outport  Port=2
  wires:
  i16_13/1 -> phase/1
  c/1 -> b17_2_/1, b33_16_/1
  ui16_16_/1 -> power/1
  b33_16_/1 -> ui16_16_/1
  b17_2_/1 -> i16_13/1

== system fftanalyzeri/c2polar_ ==
  c : Inport
  i18_15 : xbsIndex_r4/Reinterpret  force_arith_type=on  arith_type="Signed  (2's comp)"  force_bin_pt=on  bin_pt=15  block_type=reinterpret
  i18_16_ : xbsIndex_r4/Reinterpret  force_arith_type=on  arith_type="Signed  (2's comp)"  force_bin_pt=on  bin_pt=16  block_type=reinterpret
  lsb18_ : xbsIndex_r4/Slice  nbits=18  boolean_output=off  mode=Lower Bit Location + Width  bit1=0  base1=MSB of Input  bit0=0  base0=LSB of Input  dbl_ovrd=off  block_type=slice
  msb18_ : xbsIndex_r4/Slice  nbits=18  boolean_output=off  mode=Upper Bit Location + Width  bit1=0  base1=MSB of Input  bit0=0  base0=LSB of Input  dbl_ovrd=off  block_type=slice
  power : Outport
  phase : Outport  Port=2
  wires:
  i18_15/1 -> phase/1
  c/1 -> lsb18_/1, msb18_/1
  i18_16_/1 -> power/1
  msb18_/1 -> i18_16_/1
  lsb18_/1 -> i18_15/1

== system fftanalyzeri/c2polar_1 ==
  c : Inport
  i18_15 : xbsIndex_r4/Reinterpret  force_arith_type=on  arith_type="Signed  (2's comp)"  force_bin_pt=on  bin_pt=15  block_type=reinterpret
  i18_16_ : xbsIndex_r4/Reinterpret  force_arith_type=on  arith_type="Signed  (2's comp)"  force_bin_pt=on  bin_pt=16  block_type=reinterpret
  lsb18_ : xbsIndex_r4/Slice  nbits=18  boolean_output=off  mode=Lower Bit Location + Width  bit1=0  base1=MSB of Input  bit0=0  base0=LSB of Input  dbl_ovrd=off  block_type=slice
  msb18_ : xbsIndex_r4/Slice  nbits=18  boolean_output=off  mode=Upper Bit Location + Width  bit1=0  base1=MSB of Input  bit0=0  base0=LSB of Input  dbl_ovrd=off  block_type=slice
  power : Outport
  phase : Outport  Port=2
  wires:
  i18_15/1 -> phase/1
  c/1 -> lsb18_/1, msb18_/1
  i18_16_/1 -> power/1
  msb18_/1 -> i18_16_/1
  lsb18_/1 -> i18_15/1

== system fftanalyzeri/c2polar_2 ==
  c : Inport
  i18_15 : xbsIndex_r4/Reinterpret  force_arith_type=on  arith_type="Signed  (2's comp)"  force_bin_pt=on  bin_pt=15  block_type=reinterpret
  i18_16_ : xbsIndex_r4/Reinterpret  force_arith_type=on  arith_type="Signed  (2's comp)"  force_bin_pt=on  bin_pt=16  block_type=reinterpret
  lsb18_ : xbsIndex_r4/Slice  nbits=18  boolean_output=off  mode=Lower Bit Location + Width  bit1=0  base1=MSB of Input  bit0=0  base0=LSB of Input  dbl_ovrd=off  block_type=slice
  msb18_ : xbsIndex_r4/Slice  nbits=18  boolean_output=off  mode=Upper Bit Location + Width  bit1=0  base1=MSB of Input  bit0=0  base0=LSB of Input  dbl_ovrd=off  block_type=slice
  power : Outport
  phase : Outport  Port=2
  wires:
  i18_15/1 -> phase/1
  c/1 -> lsb18_/1, msb18_/1
  i18_16_/1 -> power/1
  msb18_/1 -> i18_16_/1
  lsb18_/1 -> i18_15/1

== system fftanalyzeri/c2polar_3 ==
  c : Inport
  i18_15 : xbsIndex_r4/Reinterpret  force_arith_type=on  arith_type="Signed  (2's comp)"  force_bin_pt=on  bin_pt=15  block_type=reinterpret
  i18_16_ : xbsIndex_r4/Reinterpret  force_arith_type=on  arith_type="Signed  (2's comp)"  force_bin_pt=on  bin_pt=16  block_type=reinterpret
  lsb18_ : xbsIndex_r4/Slice  nbits=18  boolean_output=off  mode=Lower Bit Location + Width  bit1=0  base1=MSB of Input  bit0=0  base0=LSB of Input  dbl_ovrd=off  block_type=slice
  msb18_ : xbsIndex_r4/Slice  nbits=18  boolean_output=off  mode=Upper Bit Location + Width  bit1=0  base1=MSB of Input  bit0=0  base0=LSB of Input  dbl_ovrd=off  block_type=slice
  power : Outport
  phase : Outport  Port=2
  wires:
  i18_15/1 -> phase/1
  c/1 -> lsb18_/1, msb18_/1
  i18_16_/1 -> power/1
  msb18_/1 -> i18_16_/1
  lsb18_/1 -> i18_15/1

== system fftanalyzeri/c2polar_5 ==
  c : Inport
  i18_15 : xbsIndex_r4/Reinterpret  force_arith_type=on  arith_type="Signed  (2's comp)"  force_bin_pt=on  bin_pt=15  block_type=reinterpret
  i18_16_ : xbsIndex_r4/Reinterpret  force_arith_type=on  arith_type="Signed  (2's comp)"  force_bin_pt=on  bin_pt=16  block_type=reinterpret
  lsb18_ : xbsIndex_r4/Slice  nbits=18  boolean_output=off  mode=Lower Bit Location + Width  bit1=0  base1=MSB of Input  bit0=0  base0=LSB of Input  dbl_ovrd=off  block_type=slice
  msb18_ : xbsIndex_r4/Slice  nbits=18  boolean_output=off  mode=Upper Bit Location + Width  bit1=0  base1=MSB of Input  bit0=0  base0=LSB of Input  dbl_ovrd=off  block_type=slice
  power : Outport
  phase : Outport  Port=2
  wires:
  i18_15/1 -> phase/1
  c/1 -> lsb18_/1, msb18_/1
  i18_16_/1 -> power/1
  msb18_/1 -> i18_16_/1
  lsb18_/1 -> i18_15/1

== system fftanalyzeri/controlReg ==
  sim_reg : Inport
  fftanalyzeri_controlReg_user_data_out : xbsIndex_r4/Gateway In  gui_display_data_type=Fixed-point  arith_type=Unsigned  n_bits=32  bin_pt=0  preci_type=Single  exp_width=8  frac_width=24  quantization="Round  (unbiased: +/- Inf)"  overflow=Saturate  period=1  dbl_ovrd=off  timing_constraint=None  locs_specified=off  LOCs={}  UseAsADC=off  ADCChannel='1'  inherit_from_input=off  hdl_port=on  block_type=gatewayin
  io_delay : xbsIndex_r4/Delay  rst=off  infoeditControl=Selection of Reset will increase slice count due to use of real FFs and instead of SRLs  en=off  latency=0  dbl_ovrd=off  reg_retiming=on  block_type=delay
  reint1 : xbsIndex_r4/Reinterpret  force_arith_type=on  arith_type=Unsigned  force_bin_pt=on  bin_pt=0  block_type=reinterpret
  slice_reg : xbsIndex_r4/Slice  nbits=32  boolean_output=off  mode=Lower Bit Location + Width  bit1=0  base1=MSB of Input  bit0=0  base0=LSB of Input  dbl_ovrd=off  block_type=slice
  in_reg : Outport
  wires:
  fftanalyzeri_controlReg_user_data_out/1 -> io_delay/1
  sim_reg/1 -> fftanalyzeri_controlReg_user_data_out/1
  io_delay/1 -> slice_reg/1
  slice_reg/1 -> reint1/1
  reint1/1 -> in_reg/1
